simulink model "Simulink_ABS_Braking_Vehicle_Dynamics"  (R2024b)
settings: Solver=VariableStepAuto  StartTime=0.0  StopTime=10.0  RelTol=1e-3
values from neighbouring files (symbols this model uses):
  delta = 5 * pi/180    (= 0.0872664625997)    [ABS_MAtlab_Script_Automation.m]
  I_w = 1.12    [ABS_MAtlab_Script_Automation.m]
  lambda_bp = (0:0.05:1)'    [ABS_MAtlab_Script_Automation.m]
  m = 1400    [ABS_MAtlab_Script_Automation.m]
  mu_dry = ([0.00  0.40  0.80  0.97  1.00  0.98  0.96  0.94  0.92  0.90 0.88  0.85  0.83  0.81  0.79  0.77  0.75  0.73  0.72  0.71  0.70 ])'    [ABS_MAtlab_Script_Automation.m]
  mu_ice = ([0.00  0.05  0.10  0.12  0.13  0.14  0.14  0.14  0.14  0.14  0.14  0.14  0.14  0.14  0.14  0.14  0.14  0.14  0.14  0.14  0.14 ])'    [ABS_MAtlab_Script_Automation.m]
  mu_wet = ([0.00  0.25  0.45  0.55  0.60  0.62  0.61  0.60  0.59  0.58 0.57  0.56  0.55  0.54  0.53  0.52  0.50  0.48  0.46  0.44  0.42 ])'    [ABS_MAtlab_Script_Automation.m]
  r = 0.33    [ABS_MAtlab_Script_Automation.m]
  T_brake = 2000    [ABS_MAtlab_Script_Automation.m]
  v0 = 100/3.6    (= 27.7777777778)    [ABS_MAtlab_Script_Automation.m]
  w0 = v0/r    (= 84.1750841751)    [ABS_MAtlab_Script_Automation.m]
libraries: simulink x8, slpidlib x4
(part 2 of 2)

== system Simulink_ABS_Braking_Vehicle_Dynamics/Braking_Without_ABS/Longitudinal_dynamics/Rear_Wheel_Right_CAlculation/angular_accelration_Wo_ABS ==
  F_x_RR : Inport
  Constant : Constant  Value=T_brake
  Constant1 : Constant  Value=r
  Constant2 : Constant  Value=I_w
  MATLAB Function1 : MATLAB Function  TreatAsAtomicUnit=on
  dw_dt : Outport
  wires:
  F_x_RR/1 -> MATLAB Function1/3(F_x_RR)
  MATLAB Function1/1(dw_dt) -> dw_dt/1
  Constant2/1 -> MATLAB Function1/4(I_w)
  Constant1/1 -> MATLAB Function1/2(r)
  Constant/1 -> MATLAB Function1/1(T_brake)

== system Simulink_ABS_Braking_Vehicle_Dynamics/Braking_Without_ABS/Longitudinal_dynamics/Rear_Wheel_left_CAlculation/Slip Calculation ==
  v : Inport
  w : Inport  Port=2
  Constant3 : Constant  Value=r
  MATLAB Function2 : MATLAB Function  TreatAsAtomicUnit=on
  lambda : Outport
  wires:
  w/1 -> MATLAB Function2/3(w)
  MATLAB Function2/1(lambda) -> lambda/1
  v/1 -> MATLAB Function2/1(v)
  Constant3/1 -> MATLAB Function2/2(r)

== system Simulink_ABS_Braking_Vehicle_Dynamics/Braking_Without_ABS/Longitudinal_dynamics/Rear_Wheel_left_CAlculation/Vehicle Speed_Block ==
  a : Inport
  Constant3 : Constant  Value=0.8
  Constant4 : Constant  Value=0.55
  Constant5 : Constant  Value=0.14
  Force_Calculation_No_ABS : MATLAB Function  TreatAsAtomicUnit=on
  MATLAB Function : MATLAB Function  TreatAsAtomicUnit=on
  Multiport Switch : MultiPortSwitch  SaturateOnIntegerOverflow=off  InputSameDT=off
  Repeating Sequence Stair : simulink/Sources/Repeating Sequence Stair  OutValues=roadSequence  tsamp=time_Road_Sequence  OutMin=[]  OutMax=[]  OutDataTypeStr=double  OutputDataTypeScalingMode=double  OutDataType=fixdt(0,8)  ConRadixGroup=Best Precision: Vector-wise  OutScaling=2^-12
  F_x_RL : Outport
  wires:
  Multiport Switch/1 -> Force_Calculation_No_ABS/1(mu)
  Repeating Sequence Stair/1 -> Multiport Switch/1
  Constant4/1 -> Multiport Switch/3
  Constant3/1 -> Multiport Switch/2
  Constant5/1 -> Multiport Switch/4
  Force_Calculation_No_ABS/1(F_x_RL) -> F_x_RL/1
  MATLAB Function/1(Fz_rl) -> Force_Calculation_No_ABS/2(F_z)
  a/1 -> MATLAB Function/1(a)

== system Simulink_ABS_Braking_Vehicle_Dynamics/Braking_Without_ABS/Longitudinal_dynamics/Rear_Wheel_left_CAlculation/angular_accelration_Wo_ABS ==
  F_x_RL : Inport
  Constant : Constant  Value=T_brake
  Constant1 : Constant  Value=r
  Constant2 : Constant  Value=I_w
  MATLAB Function1 : MATLAB Function  TreatAsAtomicUnit=on
  dw_dt : Outport
  wires:
  F_x_RL/1 -> MATLAB Function1/3(F_x_RL)
  MATLAB Function1/1(dw_dt) -> dw_dt/1
  Constant2/1 -> MATLAB Function1/4(I_w)
  Constant1/1 -> MATLAB Function1/2(r)
  Constant/1 -> MATLAB Function1/1(T_brake)

== matlab function Simulink_ABS_Braking_Vehicle_Dynamics/Braking_Without_ABS/Longitudinal_dynamics/Front_Wheel_right_CAlculation/Vehicle Speed_Block/Force_Calculation_No_ABS ==
  data: mu input; F_x_fr output; F_z input
function F_x_fr = fcn_noABS(mu, F_z)
% Computes longitudinal force per wheel without ABS

F_x_fr = mu * F_z;

end

== matlab function Simulink_ABS_Braking_Vehicle_Dynamics/Braking_Without_ABS/Longitudinal_dynamics/Front_Wheel_right_CAlculation/angular_accelration_Wo_ABS/MATLAB Function1 ==
  data: T_brake input; r input; F_x_fr input; dw_dt output; I_w input
function dw_dt = fcn(T_brake ,r, F_x_fr,I_w)

dw_dt = -(T_brake - r*F_x_fr)/I_w;

end

== matlab function Simulink_ABS_Braking_Vehicle_Dynamics/Braking_Without_ABS/Longitudinal_dynamics/Rear_Wheel_Right_CAlculation/Slip Calculation/MATLAB Function2 ==
  data: v input; r input; lambda output; w input
function lambda = fcn(v, r, w)
if v > 0.5
    lambda_raw = (v - r*w)/v;
    lambda = max(0, lambda_raw);  % clamp negative slips to 0
else
    lambda = 0;
end
end

== matlab function Simulink_ABS_Braking_Vehicle_Dynamics/Braking_Without_ABS/Longitudinal_dynamics/Front_Wheel_left_CAlculation/angular_accelration_Wo_ABS/MATLAB Function1 ==
  data: T_brake input; r input; F_x_lf input; dw_dt output; I_w input
function dw_dt = fcn(T_brake ,r, F_x_lf,I_w)

dw_dt = -(T_brake - r*F_x_lf)/I_w;

end

== matlab function Simulink_ABS_Braking_Vehicle_Dynamics/Braking_Without_ABS/Longitudinal_dynamics/Rear_Wheel_Right_CAlculation/Vehicle Speed_Block/Force_Calculation_No_ABS ==
  data: mu input; F_x_RR output; F_z input
function F_x_RR = fcn_noABS(mu, F_z)
% Computes longitudinal force per wheel without ABS

F_x_RR = mu * F_z;

end

== matlab function Simulink_ABS_Braking_Vehicle_Dynamics/Braking_Without_ABS/Longitudinal_dynamics/Rear_Wheel_Right_CAlculation/angular_accelration_Wo_ABS/MATLAB Function1 ==
  data: T_brake input; r input; F_x_RR input; dw_dt output; I_w input
function dw_dt = fcn(T_brake ,r, F_x_RR,I_w)

dw_dt = -(T_brake - r*F_x_RR)/I_w;

end

== matlab function Simulink_ABS_Braking_Vehicle_Dynamics/Braking_WIth_ABS/Longitudinal_Dynamics_ABS/ABS_Front_Right/Force_Calculation/Longitudinal force Calculation  Front ==
  data: mu_f input; F_x_fr output; F_z input; lambda_f input
function F_x_fr = fcn_front_FR(mu_f, F_z, lambda_f)
% Computes longitudinal force for front wheel using Pacejka Magic Formula
% Inputs:
%   mu_f     – Peak friction coefficient from your road lookup table
%   F_z      – Normal load on the wheel [N]
%   lambda_f – Longitudinal slip ratio

% Pacejka (Magic Formula) coefficients – generic passenger-car values
B = 10;       % stiffness factor
C = 1.9;      % shape factor
E = 0.97;     % curvature factor
D = mu_f;     % use lookup-table peak mu as the scaling factor

% Magic Formula to get effective friction coefficient mu(lambda)
mu = D * sin( C * atan( B*lambda_f - E*( B*lambda_f - atan(B*lambda_f) ) ) );

% Longitudinal tire force
F_x_fr = mu * F_z;

end

== matlab function Simulink_ABS_Braking_Vehicle_Dynamics/Braking_WIth_ABS/Longitudinal_Dynamics_ABS/ABS_Front_Right/Slip Calculation_ABS/MATLAB Function2 ==
  data: v input; r input; lambda output; w input
function lambda = fcn(v,r, w)

if v>0.2
    lambda = (v-r*w)/v ;
else
    lambda = 0 ;


end

== matlab function Simulink_ABS_Braking_Vehicle_Dynamics/Braking_WIth_ABS/Longitudinal_Dynamics_ABS/ABS_Front_Right/angular_accelration_withABS/MATLAB Function1 ==
  data: T_brake input; r input; F_x_fr input; dw_dt output; I_w input
function dw_dt = fcn(T_brake ,r, F_x_fr,I_w)

dw_dt = -(T_brake - r*F_x_fr)/I_w;

end

== matlab function Simulink_ABS_Braking_Vehicle_Dynamics/Braking_WIth_ABS/Longitudinal_Dynamics_ABS/ABS_Rear_Left/Force_Caculation/Longitudinal force Calculation  Front ==
  data: mu_f input; F_x_rl output; F_z input; lambda_f input
function F_x_rl = fcn_Rear_RL(mu_f, F_z, lambda_f)
% Computes longitudinal force for front wheel using Pacejka Magic Formula
% Inputs:
%   mu_f     – Peak friction coefficient from your road lookup table
%   F_z      – Normal load on the wheel [N]
%   lambda_f – Longitudinal slip ratio

% Pacejka (Magic Formula) coefficients – generic passenger-car values
B = 10;       % stiffness factor
C = 1.9;      % shape factor
E = 0.97;     % curvature factor
D = mu_f;     % use lookup-table peak mu as the scaling factor

% Magic Formula to get effective friction coefficient mu(lambda)
mu = D * sin( C * atan( B*lambda_f - E*( B*lambda_f - atan(B*lambda_f) ) ) );

% Longitudinal tire force
F_x_rl = mu * F_z;

end

== matlab function Simulink_ABS_Braking_Vehicle_Dynamics/Braking_WIth_ABS/Longitudinal_Dynamics_ABS/ABS_Rear_Left/Slip Calculation_ABS_rl/MATLAB Function2 ==
  data: v input; r input; lambda output; w input
function lambda = fcn(v,r, w)

if v>0.2
    lambda = (v-r*w)/v ;
else
    lambda = 0 ;


end

== matlab function Simulink_ABS_Braking_Vehicle_Dynamics/Braking_WIth_ABS/Longitudinal_Dynamics_ABS/ABS_Rear_Left/angular_accelration_withABS/MATLAB Function1 ==
  data: T_brake input; r input; F_x_rl input; dw_dt output; I_w input
function dw_dt = fcn(T_brake ,r, F_x_rl,I_w)

dw_dt = -(T_brake - r*F_x_rl)/I_w;

end

== matlab function Simulink_ABS_Braking_Vehicle_Dynamics/Braking_WIth_ABS/Longitudinal_Dynamics_ABS/ABS_Rear_Right/Force_Calculation_Rear_Right/Longitudinal force Calculation  Front ==
  data: mu_f input; F_x_rr output; F_z input; lambda_f input
function F_x_rr = fcn_Rear_RR(mu_f, F_z, lambda_f)
% Computes longitudinal force for front wheel using Pacejka Magic Formula
% Inputs:
%   mu_f     – Peak friction coefficient from your road lookup table
%   F_z      – Normal load on the wheel [N]
%   lambda_f – Longitudinal slip ratio

% Pacejka (Magic Formula) coefficients – generic passenger-car values
B = 10;       % stiffness factor
C = 1.9;      % shape factor
E = 0.97;     % curvature factor
D = mu_f;     % use lookup-table peak mu as the scaling factor

% Magic Formula to get effective friction coefficient mu(lambda)
mu = D * sin( C * atan( B*lambda_f - E*( B*lambda_f - atan(B*lambda_f) ) ) );

% Longitudinal tire force
F_x_rr = mu * F_z;

end

== matlab function Simulink_ABS_Braking_Vehicle_Dynamics/Braking_WIth_ABS/Longitudinal_Dynamics_ABS/ABS_Rear_Right/Slip Calculation_ABS_rl/MATLAB Function2 ==
  data: v input; r input; lambda output; w input
function lambda = fcn(v,r, w)

if v>0.2
    lambda = (v-r*w)/v ;
else
    lambda = 0 ;


end

== matlab function Simulink_ABS_Braking_Vehicle_Dynamics/Braking_WIth_ABS/Longitudinal_Dynamics_ABS/ABS_Rear_Right/angular_accelration_withABS/MATLAB Function1 ==
  data: T_brake input; r input; F_x_rr input; dw_dt output; I_w input
function dw_dt = fcn(T_brake ,r, F_x_rr,I_w)

dw_dt = -(T_brake - r*F_x_rr)/I_w;

end

== matlab function Simulink_ABS_Braking_Vehicle_Dynamics/Braking_Without_ABS/Longitudinal_dynamics/Rear_Wheel_left_CAlculation/Slip Calculation/MATLAB Function2 ==
  data: v input; r input; lambda output; w input
function lambda = fcn(v, r, w)
if v > 0.5
    lambda_raw = (v - r*w)/v;
    lambda = max(0, lambda_raw);  % clamp negative slips to 0
else
    lambda = 0;
end
end

== matlab function Simulink_ABS_Braking_Vehicle_Dynamics/Braking_Without_ABS/Longitudinal_dynamics/Front_Wheel_left_CAlculation/Vehicle Speed_Block/MATLAB Function ==
  data: a input; Fz_fl output
function Fz_fl = compute_dynamic_Fz(a)
% Computes dynamic normal loads per wheel during braking
% Inputs:
%   a - vehicle longitudinal acceleration [m/s^2] (negative for braking)
% Outputs:
%   Fz_fl, Fz_fr, Fz_rl, Fz_rr - normal loads per wheel [N]

%% Vehicle parameters
m   = 1400;    % vehicle mass [kg]
g   = 9.81;    % gravity [m/s^2]
h   = 0.55;    % CG height [m]
L_f = 1.1;     % distance CG to front axle [m]
L_r = 1.6;     % distance CG to rear axle [m]

%% Compute dynamic axle loads
Fz_front = (m*g*L_r - m*a*h)/(L_f + L_r);
%Fz_rear  = (m*g*L_f + m*a*h)/(L_f + L_r);

%% Divide by 2 for each wheel
Fz_fl = Fz_front / 2;
%Fz_fr = Fz_front / 2;
%Fz_rl = Fz_rear  / 2;
%Fz_rr = Fz_rear  / 2;

end

== matlab function Simulink_ABS_Braking_Vehicle_Dynamics/Braking_Without_ABS/Longitudinal_dynamics/Front_Wheel_right_CAlculation/Vehicle Speed_Block/MATLAB Function ==
  data: a input; Fz_fr output
function Fz_fr = compute_dynamic_Fz(a)
% Computes dynamic normal loads per wheel during braking
% Inputs:
%   a - vehicle longitudinal acceleration [m/s^2] (negative for braking)
% Outputs:
%   Fz_fl, Fz_fr, Fz_rl, Fz_rr - normal loads per wheel [N]

%% Vehicle parameters
m   = 1400;    % vehicle mass [kg]
g   = 9.81;    % gravity [m/s^2]
h   = 0.55;    % CG height [m]
L_f = 1.1;     % distance CG to front axle [m]
L_r = 1.6;     % distance CG to rear axle [m]

%% Compute dynamic axle loads
Fz_front = (m*g*L_r - m*a*h)/(L_f + L_r);
%Fz_rear  = (m*g*L_f + m*a*h)/(L_f + L_r);

%% Divide by 2 for each wheel
%Fz_fl = Fz_front / 2;
Fz_fr = Fz_front / 2;
%Fz_rl = Fz_rear  / 2;
%Fz_rr = Fz_rear  / 2;

end

== matlab function Simulink_ABS_Braking_Vehicle_Dynamics/Braking_Without_ABS/Longitudinal_dynamics/Rear_Wheel_left_CAlculation/Vehicle Speed_Block/MATLAB Function ==
  data: a input; Fz_rl output
function Fz_rl = compute_dynamic_Fz(a)
% Computes dynamic normal loads per wheel during braking
% Inputs:
%   a - vehicle longitudinal acceleration [m/s^2] (negative for braking)
% Outputs:
%   Fz_fl, Fz_fr, Fz_rl, Fz_rr - normal loads per wheel [N]

%% Vehicle parameters
m   = 1400;    % vehicle mass [kg]
g   = 9.81;    % gravity [m/s^2]
h   = 0.55;    % CG height [m]
L_f = 1.1;     % distance CG to front axle [m]
L_r = 1.6;     % distance CG to rear axle [m]

%% Compute dynamic axle loads
%Fz_front = (m*g*L_r - m*a*h)/(L_f + L_r);
Fz_rear  = (m*g*L_f + m*a*h)/(L_f + L_r);

%% Divide by 2 for each wheel
%Fz_fl = Fz_front / 2;
%Fz_fr = Fz_front / 2;
Fz_rl = Fz_rear  / 2;
%Fz_rr = Fz_rear  / 2;

end

== matlab function Simulink_ABS_Braking_Vehicle_Dynamics/Braking_Without_ABS/Longitudinal_dynamics/Rear_Wheel_Right_CAlculation/Vehicle Speed_Block/MATLAB Function ==
  data: a input; Fz_rr output
function Fz_rr = compute_dynamic_Fz(a)
% Computes dynamic normal loads per wheel during braking
% Inputs:
%   a - vehicle longitudinal acceleration [m/s^2] (negative for braking)
% Outputs:
%   Fz_fl, Fz_fr, Fz_rl, Fz_rr - normal loads per wheel [N]

%% Vehicle parameters
m   = 1400;    % vehicle mass [kg]
g   = 9.81;    % gravity [m/s^2]
h   = 0.55;    % CG height [m]
L_f = 1.1;     % distance CG to front axle [m]
L_r = 1.6;     % distance CG to rear axle [m]

%% Compute dynamic axle loads
%Fz_front = (m*g*L_r - m*a*h)/(L_f + L_r);
Fz_rear  = (m*g*L_f + m*a*h)/(L_f + L_r);

%% Divide by 2 for each wheel
%Fz_fl = Fz_front / 2;
%Fz_fr = Fz_front / 2;
%Fz_rl = Fz_rear  / 2;
Fz_rr = Fz_rear  / 2;

end

== matlab function Simulink_ABS_Braking_Vehicle_Dynamics/Braking_WIth_ABS/Longitudinal_Dynamics_ABS/ABS_Front_LEFT/Force_Calculation/MATLAB Function ==
  data: a input; Fz_fl output
function Fz_fl = compute_dynamic_Fz(a)
% Computes dynamic normal loads per wheel during braking
% Inputs:
%   a - vehicle longitudinal acceleration [m/s^2] (negative for braking)
% Outputs:
%   Fz_fl, Fz_fr, Fz_rl, Fz_rr - normal loads per wheel [N]

%% Vehicle parameters
m   = 1400;    % vehicle mass [kg]
g   = 9.81;    % gravity [m/s^2]
h   = 0.55;    % CG height [m]
L_f = 1.1;     % distance CG to front axle [m]
L_r = 1.6;     % distance CG to rear axle [m]

%% Compute dynamic axle loads
Fz_front = (m*g*L_r - m*a*h)/(L_f + L_r);
%Fz_rear  = (m*g*L_f + m*a*h)/(L_f + L_r);

%% Divide by 2 for each wheel
Fz_fl = Fz_front / 2;
%Fz_fr = Fz_front / 2;
%Fz_rl = Fz_rear  / 2;
%Fz_rr = Fz_rear  / 2;

end

== matlab function Simulink_ABS_Braking_Vehicle_Dynamics/Braking_WIth_ABS/Longitudinal_Dynamics_ABS/ABS_Front_Right/Force_Calculation/MATLAB Function ==
  data: a input; Fz_fr output
function Fz_fr = compute_dynamic_Fz(a)
% Computes dynamic normal loads per wheel during braking
% Inputs:
%   a - vehicle longitudinal acceleration [m/s^2] (negative for braking)
% Outputs:
%   Fz_fl, Fz_fr, Fz_rl, Fz_rr - normal loads per wheel [N]

%% Vehicle parameters
m   = 1400;    % vehicle mass [kg]
g   = 9.81;    % gravity [m/s^2]
h   = 0.55;    % CG height [m]
L_f = 1.1;     % distance CG to front axle [m]
L_r = 1.6;     % distance CG to rear axle [m]

%% Compute dynamic axle loads
Fz_front = (m*g*L_r - m*a*h)/(L_f + L_r);
%Fz_rear  = (m*g*L_f + m*a*h)/(L_f + L_r);

%% Divide by 2 for each wheel
%Fz_fl = Fz_front / 2;
Fz_fr = Fz_front / 2;
%Fz_rl = Fz_rear  / 2;
%Fz_rr = Fz_rear  / 2;

end

== matlab function Simulink_ABS_Braking_Vehicle_Dynamics/Braking_WIth_ABS/Longitudinal_Dynamics_ABS/ABS_Rear_Left/Force_Caculation/MATLAB Function ==
  data: a input; Fz_rl output
function Fz_rl = compute_dynamic_Fz(a)
% Computes dynamic normal loads per wheel during braking
% Inputs:
%   a - vehicle longitudinal acceleration [m/s^2] (negative for braking)
% Outputs:
%   Fz_fl, Fz_fr, Fz_rl, Fz_rr - normal loads per wheel [N]

%% Vehicle parameters
m   = 1400;    % vehicle mass [kg]
g   = 9.81;    % gravity [m/s^2]
h   = 0.55;    % CG height [m]
L_f = 1.1;     % distance CG to front axle [m]
L_r = 1.6;     % distance CG to rear axle [m]

%% Compute dynamic axle loads
%Fz_front = (m*g*L_r - m*a*h)/(L_f + L_r);
Fz_rear  = (m*g*L_f + m*a*h)/(L_f + L_r);

%% Divide by 2 for each wheel
%Fz_fl = Fz_front / 2;
%Fz_fr = Fz_front / 2;
Fz_rl = Fz_rear  / 2;
%Fz_rr = Fz_rear  / 2;

end

== matlab function Simulink_ABS_Braking_Vehicle_Dynamics/Braking_WIth_ABS/Longitudinal_Dynamics_ABS/ABS_Rear_Right/Force_Calculation_Rear_Right/MATLAB Function ==
  data: a input; Fz_rr output
function Fz_rr = compute_dynamic_Fz(a)
% Computes dynamic normal loads per wheel during braking
% Inputs:
%   a - vehicle longitudinal acceleration [m/s^2] (negative for braking)
% Outputs:
%   Fz_fl, Fz_fr, Fz_rl, Fz_rr - normal loads per wheel [N]

%% Vehicle parameters
m   = 1400;    % vehicle mass [kg]
g   = 9.81;    % gravity [m/s^2]
h   = 0.55;    % CG height [m]
L_f = 1.1;     % distance CG to front axle [m]
L_r = 1.6;     % distance CG to rear axle [m]

%% Compute dynamic axle loads
%Fz_front = (m*g*L_r - m*a*h)/(L_f + L_r);
Fz_rear  = (m*g*L_f + m*a*h)/(L_f + L_r);

%% Divide by 2 for each wheel
%Fz_fl = Fz_front / 2;
%Fz_fr = Fz_front / 2;
%Fz_rl = Fz_rear  / 2;
Fz_rr = Fz_rear  / 2;

end

== matlab function Simulink_ABS_Braking_Vehicle_Dynamics/Braking_Without_ABS/Lateral_Dynamics/MATLAB Function ==
  data: V_x input; V_y input; r input; Fy_f output; delta input; Fy_r output
function [Fy_f, Fy_r] = fcn_lateral(V_x, V_y, r, delta)
% Computes front and rear axle lateral forces using a linear bicycle model

%% Vehicle parameters
a = 1.1;       
b = 1.6;       
I_z = 1500;    
m = 1400;      
C_f = 60000;   
C_r = 60000;   

%% Minimum speed threshold to avoid division by zero
Vx_min = 0.3;  % m/s
if V_x < Vx_min
    Fy_f = 0;
    Fy_r = 0;
    return
end

%% Compute lateral forces
Fy_f = C_f * (delta - (V_y + a*r)/V_x);
Fy_r = C_r * (-(V_y - b*r)/V_x);

end

== matlab function Simulink_ABS_Braking_Vehicle_Dynamics/Braking_Without_ABS/Lateral_Dynamics/MATLAB Function1 ==
  data: Fy_f input; dy_dt output; Fy_r input; V_x input; r input; dr_dt output
function [dy_dt, dr_dt] = fcn_bicycle(Fy_f, Fy_r, V_x,  r)
% Computes lateral and yaw acceleration for a bicycle model
%
% Inputs:
%   Fy_f - front axle lateral force [N]
%   Fy_r - rear axle lateral force [N]
%   V_x  - longitudinal velocity [m/s]
%   V_y  - lateral velocity [m/s]
%   r    - yaw rate [rad/s]
%
% Outputs:
%   dy_dt - lateral acceleration [m/s^2]
%   dr_dt - yaw acceleration [rad/s^2]

%% Vehicle parameters
m = 1400;      % mass [kg]
a = 1.1;       % CG to front axle [m]
b = 1.6;       % CG to rear axle [m]
I_z = 1500;    % yaw inertia [kg*m^2]

%% Avoid calculation if vehicle stopped
if V_x <= 0
    dy_dt = 0;
    dr_dt = 0;
    return
end

%% Lateral acceleration
dy_dt = (Fy_f + Fy_r)/m - V_x*r;

%% Yaw acceleration
dr_dt = (a*Fy_f - b*Fy_r)/I_z;

end

== matlab function Simulink_ABS_Braking_Vehicle_Dynamics/Braking_WIth_ABS/Usage_ECS_Monitoring/Front_Left Wheel/MATLAB Function ==
  data: Fx input; Fy input; Fz input; mu input; usage_FL output
function  usage_FL = fcn_friction_usage(Fx, Fy, Fz, mu)
% Computes tire friction usage using simple threshold logic

% Thresholds
Fz_min = 0.2;   % minimum wheel load [N] to consider
mu_min = 0.2;   % minimum friction coefficient

if Fz > Fz_min && mu > mu_min
    limit = mu * Fz;                     % available friction
    usage_FL = sqrt(Fx^2 + Fy^2)/limit;     % normalized usage
else
    usage_FL = 0;                            % ignore tiny load / mu
  
end



end

== matlab function Simulink_ABS_Braking_Vehicle_Dynamics/Braking_Without_ABS/Longitudinal_dynamics/Front_Wheel_left_CAlculation/Slip Calculation/MATLAB Function2 ==
  data: v input; r input; lambda output; w_lf input
function lambda = fcn(v, r, w_lf)
if v > 0.5
    lambda_raw = (v - r*w_lf)/v;
    lambda = max(0, lambda_raw);  % clamp negative slips to 0
else
    lambda = 0;
end
end

== matlab function Simulink_ABS_Braking_Vehicle_Dynamics/Braking_WIth_ABS/Lateral_Dynamics_ABS/MATLAB Function ==
  data: V_x input; V_y input; r input; Fy_f output; delta input; Fy_r output
function [Fy_f, Fy_r] = fcn_lateral(V_x, V_y, r, delta)
% Computes front and rear axle lateral forces using a linear bicycle model

%% Vehicle parameters
a = 1.1;       
b = 1.6;       
I_z = 1500;    
m = 1400;      
C_f = 60000;   
C_r = 60000;   

%% Minimum speed threshold to avoid division by zero
Vx_min = 0.3;  % m/s
if V_x < Vx_min
    Fy_f = 0;
    Fy_r = 0;
    return
end

%% Compute lateral forces
Fy_f = C_f * (delta - (V_y + a*r)/V_x);
Fy_r = C_r * (-(V_y - b*r)/V_x);

end

== matlab function Simulink_ABS_Braking_Vehicle_Dynamics/Braking_WIth_ABS/Lateral_Dynamics_ABS/MATLAB Function1 ==
  data: Fy_f input; dy_dt output; Fy_r input; V_x input; r input; dr_dt output
function [dy_dt, dr_dt] = fcn_bicycle(Fy_f, Fy_r, V_x,  r)
% Computes lateral and yaw acceleration for a bicycle model
%
% Inputs:
%   Fy_f - front axle lateral force [N]
%   Fy_r - rear axle lateral force [N]
%   V_x  - longitudinal velocity [m/s]
%   V_y  - lateral velocity [m/s]
%   r    - yaw rate [rad/s]
%
% Outputs:
%   dy_dt - lateral acceleration [m/s^2]
%   dr_dt - yaw acceleration [rad/s^2]

%% Vehicle parameters
m = 1400;      % mass [kg]
a = 1.1;       % CG to front axle [m]
b = 1.6;       % CG to rear axle [m]
I_z = 1500;    % yaw inertia [kg*m^2]

%% Avoid calculation if vehicle stopped
if V_x <= 0
    dy_dt = 0;
    dr_dt = 0;
    return
end

%% Lateral acceleration
dy_dt = (Fy_f + Fy_r)/m - V_x*r;

%% Yaw acceleration
dr_dt = (a*Fy_f - b*Fy_r)/I_z;

end

== matlab function Simulink_ABS_Braking_Vehicle_Dynamics/Braking_WIth_ABS/Longitudinal_Dynamics_ABS/ABS_Front_LEFT/angular_accelration_withABS/MATLAB Function ==
  data: T_brake_PID input; T_brake_mod output; usage input
function T_brake_mod = fcn_abs_mod(T_brake_PID, usage)
% Brake torque modulation to keep tire usage within friction circle
%
% Inputs:
%   T_brake_PID - torque demand from PID controller [Nm]
%   usage       - tire friction usage (Fx^2+Fy^2)/(mu*Fz)^2
%
% Output:
%   T_brake_mod - adjusted brake torque [Nm]

% ---- Parameters ----
target_usage = 1.0;   % max allowed usage (set 0.9–1.0 safe)
K_mod        = 1.0;   % aggressiveness of modulation

% ---- Logic ----
if usage > target_usage
    % Scale torque down proportional to usage
    T_brake_mod = T_brake_PID * (target_usage / usage);
else
    % Pass torque unchanged
    T_brake_mod = T_brake_PID;
end

% Safety clamp: torque cannot be negative
T_brake_mod = max(T_brake_mod, 0);

end

== matlab function Simulink_ABS_Braking_Vehicle_Dynamics/Braking_WIth_ABS/Usage_ECS_Monitoring/Front_Right_Wheel/MATLAB Function ==
  data: Fx input; Fy input; Fz input; mu input; usage_FL output
function  usage_FL = fcn_friction_usage(Fx, Fy, Fz, mu)
% Computes tire friction usage using simple threshold logic

% Thresholds
Fz_min = 0.2;   % minimum wheel load [N] to consider
mu_min = 0.2;   % minimum friction coefficient

if Fz > Fz_min && mu > mu_min
    limit = mu * Fz;                     % available friction
    usage_FL = sqrt(Fx^2 + Fy^2)/limit;     % normalized usage
else
    usage_FL = 0;                            % ignore tiny load / mu
  
end



end

== matlab function Simulink_ABS_Braking_Vehicle_Dynamics/Braking_WIth_ABS/Longitudinal_Dynamics_ABS/ABS_Front_Right/angular_accelration_withABS/MATLAB Function ==
  data: T_brake_PID input; T_brake_mod output; usage input
function T_brake_mod = fcn_abs_mod(T_brake_PID, usage)
% Brake torque modulation to keep tire usage within friction circle
%
% Inputs:
%   T_brake_PID - torque demand from PID controller [Nm]
%   usage       - tire friction usage (Fx^2+Fy^2)/(mu*Fz)^2
%
% Output:
%   T_brake_mod - adjusted brake torque [Nm]

% ---- Parameters ----
target_usage = 1.0;   % max allowed usage (set 0.9–1.0 safe)
K_mod        = 1.0;   % aggressiveness of modulation

% ---- Logic ----
if usage > target_usage
    % Scale torque down proportional to usage
    T_brake_mod = T_brake_PID * (target_usage / usage);
else
    % Pass torque unchanged
    T_brake_mod = T_brake_PID;
end

% Safety clamp: torque cannot be negative
T_brake_mod = max(T_brake_mod, 0);

end

== matlab function Simulink_ABS_Braking_Vehicle_Dynamics/Braking_WIth_ABS/Usage_ECS_Monitoring/Rear_Left_Wheel/MATLAB Function ==
  data: Fx input; Fy input; Fz input; mu input; usage_FL output
function  usage_FL = fcn_friction_usage(Fx, Fy, Fz, mu)
% Computes tire friction usage using simple threshold logic

% Thresholds
Fz_min = 0.2;   % minimum wheel load [N] to consider
mu_min = 0.2;   % minimum friction coefficient

if Fz > Fz_min && mu > mu_min
    limit = mu * Fz;                     % available friction
    %Fx =0.4*Fx ;
     %Fy = 0.4*Fy ;
    usage_FL = sqrt(Fx^2 + Fy^2)/limit;     % normalized usage
else
    usage_FL = 0;                            % ignore tiny load / mu
  
end



end

== matlab function Simulink_ABS_Braking_Vehicle_Dynamics/Braking_WIth_ABS/Usage_ECS_Monitoring/Rear_Right_Wheel/MATLAB Function ==
  data: Fx input; Fy input; Fz input; mu input; usage_FL output
function  usage_FL = fcn_friction_usage(Fx, Fy, Fz, mu)
% Computes tire friction usage using simple threshold logic

% Thresholds
Fz_min = 0.2;   % minimum wheel load [N] to consider
mu_min = 0.2;   % minimum friction coefficient

if Fz > Fz_min && mu > mu_min
    limit = mu * Fz;                     % available friction
    %Fx =0.4*Fx ;
     %Fy = 0.4*Fy ;
    usage_FL = sqrt(Fx^2 + Fy^2)/limit;     % normalized usage
else
    usage_FL = 0;                            % ignore tiny load / mu
  
end



end

== matlab function Simulink_ABS_Braking_Vehicle_Dynamics/Braking_WIth_ABS/Longitudinal_Dynamics_ABS/ABS_Rear_Left/angular_accelration_withABS/MATLAB Function ==
  data: T_brake_PID input; T_brake_mod output; usage input
function T_brake_mod = fcn_abs_mod(T_brake_PID, usage)
% Brake torque modulation to keep tire usage within friction circle
%
% Inputs:
%   T_brake_PID - torque demand from PID controller [Nm]
%   usage       - tire friction usage (Fx^2+Fy^2)/(mu*Fz)^2
%
% Output:
%   T_brake_mod - adjusted brake torque [Nm]

% ---- Parameters ----
target_usage = 1.0;   % max allowed usage (set 0.9–1.0 safe)
K_mod        = 1.0;   % aggressiveness of modulation

% ---- Logic ----
if usage > target_usage
    % Scale torque down proportional to usage
    T_brake_mod = T_brake_PID * (target_usage / usage);
else
    % Pass torque unchanged
    T_brake_mod = T_brake_PID;
end

% Safety clamp: torque cannot be negative
T_brake_mod = max(T_brake_mod, 0);

end

== matlab function Simulink_ABS_Braking_Vehicle_Dynamics/Braking_WIth_ABS/Longitudinal_Dynamics_ABS/ABS_Rear_Right/angular_accelration_withABS/MATLAB Function ==
  data: T_brake_PID input; T_brake_mod output; usage input
function T_brake_mod = fcn_abs_mod(T_brake_PID, usage)
% Brake torque modulation to keep tire usage within friction circle
%
% Inputs:
%   T_brake_PID - torque demand from PID controller [Nm]
%   usage       - tire friction usage (Fx^2+Fy^2)/(mu*Fz)^2
%
% Output:
%   T_brake_mod - adjusted brake torque [Nm]

% ---- Parameters ----
target_usage = 1.0;   % max allowed usage (set 0.9–1.0 safe)
K_mod        = 1.0;   % aggressiveness of modulation

% ---- Logic ----
if usage > target_usage
    % Scale torque down proportional to usage
    T_brake_mod = T_brake_PID * (target_usage / usage);
else
    % Pass torque unchanged
    T_brake_mod = T_brake_PID;
end

% Safety clamp: torque cannot be negative
T_brake_mod = max(T_brake_mod, 0);

end

== matlab function Simulink_ABS_Braking_Vehicle_Dynamics/Braking_WIth_ABS/Longitudinal_Dynamics_ABS/ABS_Front_LEFT/angular_accelration_withABS/MATLAB Function1 ==
  data: T_brake input; r input; F_x_lf input; dw_dt output; I_w input
function dw_dt = fcn(T_brake ,r, F_x_lf,I_w)

dw_dt = -(T_brake - r*F_x_lf)/I_w;

end

== matlab function Simulink_ABS_Braking_Vehicle_Dynamics/Braking_WIth_ABS/Longitudinal_Dynamics_ABS/ABS_Front_LEFT/Slip Calculation_ABS/MATLAB Function2 ==
  data: v input; r input; lambda output; w input
function lambda = fcn(v,r, w)

if v>0.2
    lambda = (v-r*w)/v ;
else
    lambda = 0 ;


end

== matlab function Simulink_ABS_Braking_Vehicle_Dynamics/Braking_Without_ABS/Longitudinal_dynamics/Rear_Wheel_left_CAlculation/Vehicle Speed_Block/Force_Calculation_No_ABS ==
  data: mu input; F_x_RL output; F_z input
function F_x_RL = fcn_noABS(mu, F_z)
% Computes longitudinal force per wheel without ABS

F_x_RL = mu * F_z;

end

== matlab function Simulink_ABS_Braking_Vehicle_Dynamics/Braking_WIth_ABS/Longitudinal_Dynamics_ABS/ABS_Front_LEFT/Force_Calculation/Longitudinal force Calculation  Front ==
  data: mu_f input; F_x_fl output; F_z input; lambda_f input
function F_x_fl = fcn_front_FL(mu_f, F_z, lambda_f)
% Computes longitudinal force for front wheel using Pacejka Magic Formula
% Inputs:
%   mu_f     – Peak friction coefficient from your road lookup table
%   F_z      – Normal load on the wheel [N]
%   lambda_f – Longitudinal slip ratio

% Pacejka (Magic Formula) coefficients – generic passenger-car values
B = 10;       % stiffness factor
C = 1.9;      % shape factor
E = 0.97;     % curvature factor
D = mu_f;     % use lookup-table peak mu as the scaling factor

% Magic Formula to get effective friction coefficient mu(lambda)
mu = D * sin( C * atan( B*lambda_f - E*( B*lambda_f - atan(B*lambda_f) ) ) );

% Longitudinal tire force
F_x_fl = mu * F_z;

end

== matlab function Simulink_ABS_Braking_Vehicle_Dynamics/Braking_Without_ABS/Longitudinal_dynamics/Rear_Wheel_left_CAlculation/angular_accelration_Wo_ABS/MATLAB Function1 ==
  data: T_brake input; r input; F_x_RL input; dw_dt output; I_w input
function dw_dt = fcn(T_brake ,r, F_x_RL,I_w)

dw_dt = -(T_brake - r*F_x_RL)/I_w;

end

== matlab function Simulink_ABS_Braking_Vehicle_Dynamics/Braking_Without_ABS/Longitudinal_dynamics/Front_Wheel_right_CAlculation/Slip Calculation/MATLAB Function2 ==
  data: v input; r input; lambda output; w input
function lambda = fcn(v, r, w)
if v > 0.5
    lambda_raw = (v - r*w)/v;
    lambda = max(0, lambda_raw);  % clamp negative slips to 0
else
    lambda = 0;
end
end

== matlab function Simulink_ABS_Braking_Vehicle_Dynamics/Braking_Without_ABS/Longitudinal_dynamics/Front_Wheel_left_CAlculation/Vehicle Speed_Block/Force_Calculation_No_ABS ==
  data: mu input; F_x_fl output; F_z input
function F_x_fl = fcn_noABS(mu, F_z)
% Computes longitudinal force per wheel without ABS

F_x_fl = mu * F_z;

end
